simulink model "position_control"  (R2023a)
settings: Solver=VariableStepAuto  StartTime=0.0  StopTime=10.0  RelTol=1e-3
values from neighbouring files (symbols this model uses):
  K = 2.6    [Runposition_control.m]
  Ki = .1    (= 0.1)    [Runposition_control.m]
  Kp = 1.5    [Runposition_control.m]
  sigma = 9    [Runposition_control.m]
libraries: simulink x1
settings Model: Creator=small  LastModifiedBy=small

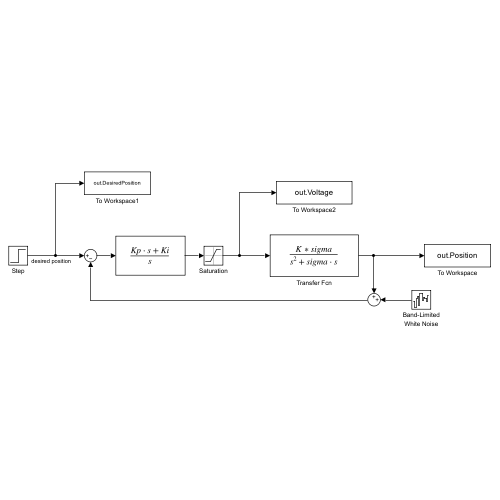
[thumbnail: Simulink's stored preview of the top-level diagram]
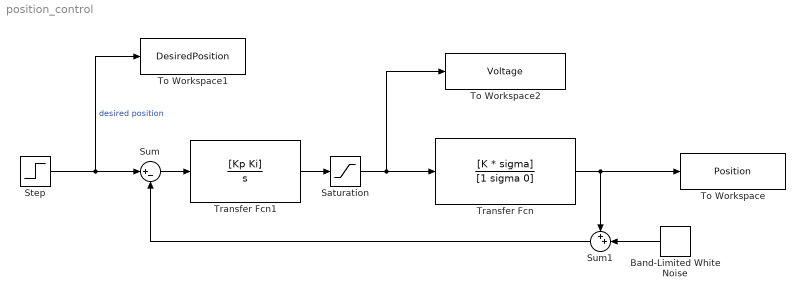
== system position_control ==
  Band-Limited White Noise : simulink/Sources/Band-Limited White Noise  Cov=[0.0001]  Ts=0.01  seed=[23341]
  Saturation : Saturate  UpperLimit=7.5  LowerLimit=-7.5
  Step : Step  After=3.141592  SampleTime=0
  Sum : Sum  Inputs=|+-
  Sum1 : Sum  Inputs=++|
  To Workspace : ToWorkspace  VariableName=Position  SaveFormat=Timeseries  SampleTime=-1
  To Workspace1 : ToWorkspace  VariableName=DesiredPosition  SaveFormat=Timeseries  SampleTime=-1
  To Workspace2 : ToWorkspace  VariableName=Voltage  SaveFormat=Timeseries  SampleTime=-1
  Transfer Fcn : TransferFcn  Numerator=[K * sigma]  Denominator=[1 sigma 0]
  Transfer Fcn1 : TransferFcn  Numerator=[Kp Ki]  Denominator=[1 0]
  wires:
  Transfer Fcn1/1 -> Saturation/1
  Sum/1 -> Transfer Fcn1/1
  Transfer Fcn/1 -> Sum1/1, To Workspace/1
  Step/1 -> To Workspace1/1, Sum/1  "desired position"
  Band-Limited White Noise/1 -> Sum1/2
  Sum1/1 -> Sum/2
  Saturation/1 -> To Workspace2/1, Transfer Fcn/1
